simulink model "PI"  (R2018b)
settings: Solver=FixedStepAuto  StartTime=0.0  StopTime=10  FixedStep=0.0005  RelTol=1e-3
values from neighbouring files (symbols this model uses):
  K1 = [0.827079899876 1.7007512609 0.705017257417 0.414213562373]    [dulieu.mat]    (also in pi2.mat; pi3.mat)
undefined symbols (not defined in the file or in its folder): K5
settings Model: Creator=User  LastModifiedBy=User

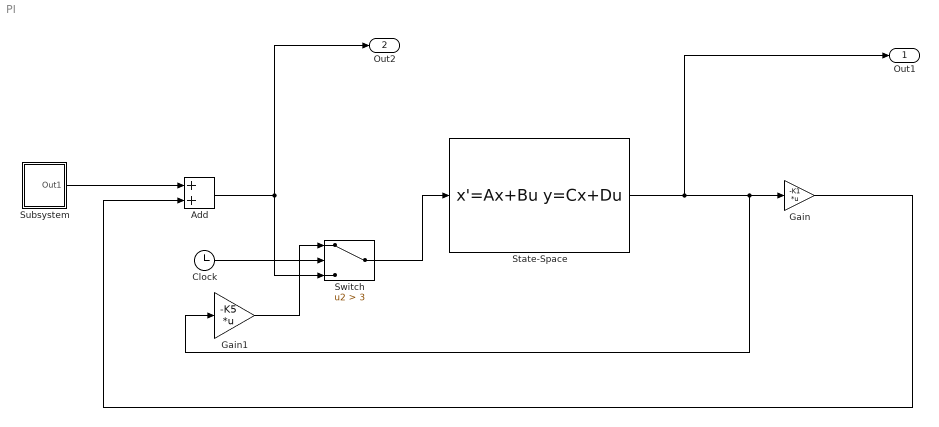
== system PI ==
  Add : Sum
  Clock : Clock
  Gain : Gain  Gain=-K1  Multiplication=Matrix(K*u)
  Gain1 : Gain  Gain=-K5  Multiplication=Matrix(K*u)
  State-Space : StateSpace  A=[-0.0665 11.5 0 0;0 -2.5 2.5 0;-9.5 0 -13.736 -13.736;0.6 0 0 0]  B=[0;0;13.736;0]  C=eye(4)  D=[0;0;0;0]  InitialCondition=[0;0.1;0;0]
  Subsystem : Subsystem
  Switch : Switch  Criteria=u2 > Threshold  Threshold=3
  Out1 : Outport
  Out2 : Outport  Port=2
  wires:
  State-Space/1 -> Gain1/1, Gain/1, Out1/1
  Add/1 -> Switch/3, Out2/1
  Subsystem/1(Out1) -> Add/1
  Gain/1 -> Add/2
  Switch/1 -> State-Space/1
  Clock/1 -> Switch/2
  Gain1/1 -> Switch/1

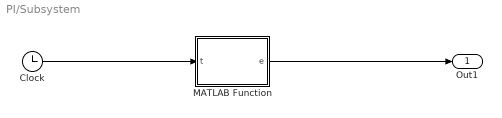
== system PI/Subsystem ==
  Clock : Clock
  MATLAB Function : MATLAB Function  TreatAsAtomicUnit=on
  Out1 : Outport
  wires:
  Clock/1 -> MATLAB Function/1(t)
  MATLAB Function/1(e) -> Out1/1

== matlab function PI/Subsystem/MATLAB Function ==
  data: t input; e output
function e = fcn(t)
w=[111.1412
   11.2334
    5.0726
  -64.4173
   -2.6645
   29.7744
   42.9925
  -25.0763
  -31.8152
  117.1157
 -110.9427
   92.4403
   99.1888
   71.0841
  -96.3091
  -57.1509
  -39.5144
   43.1347
  -87.2272
   53.0946
  -94.3772
   36.9018
   -1.3983
   66.9724
   51.6089
   96.8929
   93.8214
  -39.8009
   47.6990
  -72.5256
 -112.6702
   58.5778
    0.0054
   -4.8187
   97.1333
   26.3680
   28.2399
   86.2662
   73.3175
   18.4132
  -76.0986
  -62.4163
   92.7629
 -113.1182
   -2.4237
  -79.6975
  114.8834
   51.0467
    0.1132
   -6.9388
 -105.6915
   43.6733
 -109.8165
 -102.8531
    5.1960
  -96.7848
   76.3557
   76.2113
   53.3855
  -84.0323
   38.3053
    4.4628
  113.5139
   35.7580
   72.0793
  -11.0885
  -16.2260
   78.0753
  -99.9672
  -88.0390
  -78.3867
  -26.1749
   79.5311
   72.8075
 -105.4869
  -24.1781
    6.4502
  -19.9681
   37.6464
   30.7136
  -49.9238
  -16.4037
 -116.2831
  116.1753
  -79.8796
  -94.5081
  -30.6217
  -72.4516
   -2.4750
  -38.5216
  108.3913
  100.8797
 -107.3575
   57.0859
  -55.4113
  -18.5195
   11.4890
  106.2569
  -19.7414
  115.9326];
e=0;
for i=1:100
    e=e+0.001*sin(w(i)*t);
end
